simulink model "Planta1_simulink"  (R2023a)
settings: Solver=VariableStepAuto  StartTime=0.0  StopTime=10  MaxStep=0.001  RelTol=1e-3
settings Model: Creator=Ronny  LastModifiedBy=Ronny

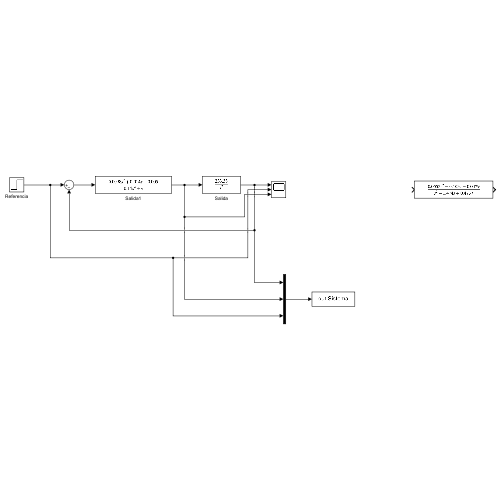
[thumbnail: Simulink's stored preview of the top-level diagram]
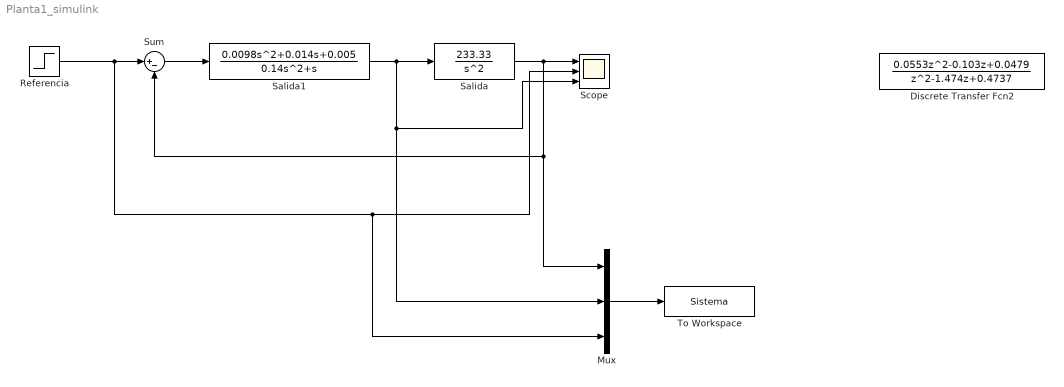
== system Planta1_simulink ==
  Discrete Transfer Fcn2 : DiscreteTransferFcn  Numerator=[0.0553 -0.103 0.0479]  Denominator=[1 -1.474 0.4737]  SampleTime=0.1
  Mux : Mux  Inputs=3
  Referencia : Step  SampleTime=0.1
  Salida : TransferFcn  Numerator=[233.33]  Denominator=[1 0 0]
  Salida1 : TransferFcn  Numerator=[0.0098 0.014 0.005]  Denominator=[0.14 1 0]
  Scope : Scope  NumInputPorts=3
  Sum : Sum  Inputs=|+-
  To Workspace : ToWorkspace  VariableName=Sistema  SaveFormat=Timeseries  SampleTime=-1
  wires:
  Salida/1 -> Mux/1, Sum/2, Scope/1
  Referencia/1 -> Mux/3, Scope/2, Sum/1
  Sum/1 -> Salida1/1
  Salida1/1 -> Scope/3, Mux/2, Salida/1
  Mux/1 -> To Workspace/1
